simulink model "SVPWM"  (R2026a)
settings: Solver=VariableStepAuto  StopTime=2
undefined symbols (not defined in the file): Down, Up
libraries: eePwmGenerator x3, simulink x3, autolibpmsminterior x2
settings Model: Creator=mushen  LastModifiedBy=mushen

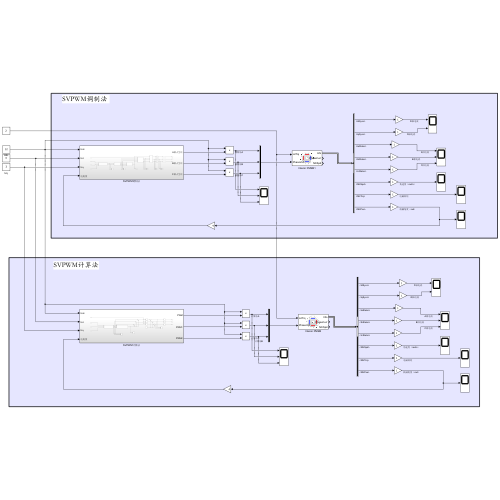
[thumbnail: Simulink's stored preview of the top-level diagram]
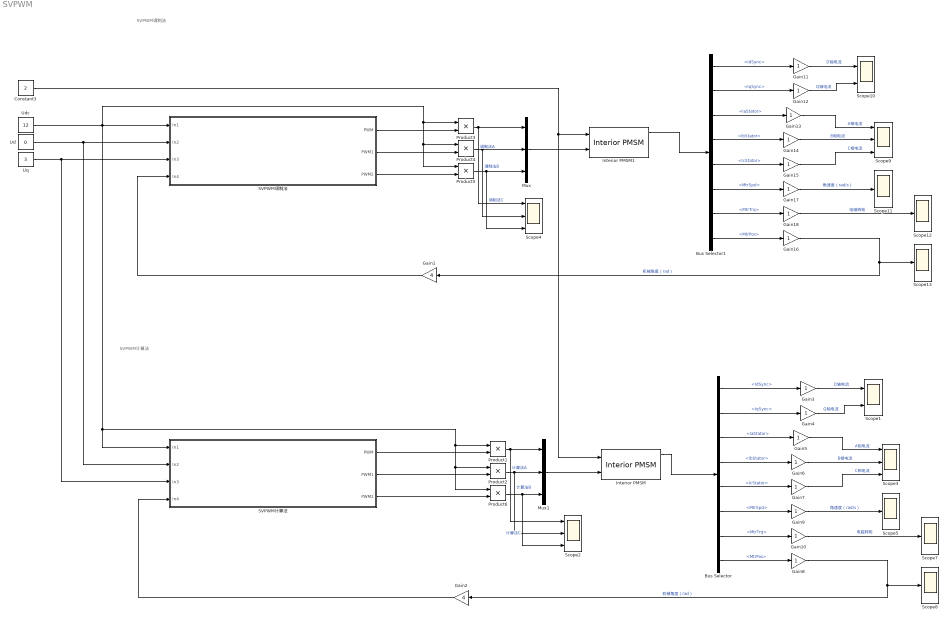
== system SVPWM ==
  note: SVPWM计算法
  note: SVPWM调制法
  Bus Selector : BusSelector  OutputSignals=IdSync,IqSync,IaStator,IbStator,IcStator,MtrSpd,MtrTrq,MtrPos
  Bus Selector1 : BusSelector  OutputSignals=IdSync,IqSync,IaStator,IbStator,IcStator,MtrSpd,MtrTrq,MtrPos
  Constant3 : Constant  Value=2
  Gain1 : Gain  Gain=4
  Gain{3..18} (16 alike) : Gain
  Gain2 : Gain  Gain=4
  Interior PMSM : autolibpmsminterior/Interior PMSM  port_config=Torque  sim_type=Continuous  Ts=0.001  P=4  Rs=0.02  Ldq=[1.7e-3 3.2e-3]  KConstText=Permanent flux linkage constant (lambda_pm):  lambda_pm=0.2205  Ke=159.9771  mechanical=[0.002700,4.924e-4,0]  idq0=[0 0]  theta_init=0  omega_init=0  KConst=0.2205  lambda_pm_calc=0.2205  Kt=0.07  RefBlkName='autolibpmsminterior/Interior PMSM'  aMode=5
      settings: LibrarySourceBlock=mcblib/Electrical Systems/Motors/Interior PMSM
  Interior PMSM1 : autolibpmsminterior/Interior PMSM  port_config=Torque  sim_type=Continuous  Ts=0.001  P=4  Rs=0.02  Ldq=[1.7e-3 3.2e-3]  KConstText=Permanent flux linkage constant (lambda_pm):  lambda_pm=0.2205  Ke=159.9771  mechanical=[0.002700,4.924e-4,0]  idq0=[0 0]  theta_init=0  omega_init=0  KConst=0.2205  lambda_pm_calc=0.2205  Kt=0.07  RefBlkName='autolibpmsminterior/Interior PMSM'  aMode=5
      settings: LibrarySourceBlock=mcblib/Electrical Systems/Motors/Interior PMSM
  Mux : Mux  Inputs=3
  Mux1 : Mux  Inputs=3
  Product{1..6} (6 alike) : Product
  SVPWM计算法 : Subsystem
  SVPWM调制法 : Subsystem
  Scope1 : Scope  NumInputPorts=2
      settings: ActiveDisplayYMinimum=-7.4999999999542695  ActiveDisplayYMaximum=7.49999999991693
  Scope10 : Scope  NumInputPorts=2
      settings: ActiveDisplayYMinimum=-7.4999999999542695  ActiveDisplayYMaximum=7.49999999991693  DataLoggingVariableName=ScopeData15
  Scope{5,7..8,11..13} (6 alike) : Scope
      Scope11 settings: ActiveDisplayYMinimum=-8.3500269440904287  ActiveDisplayYMaximum=20.77178175547505  DataLoggingVariableName=ScopeData16
      Scope12 settings: ActiveDisplayYMinimum=-7.4999999999542695  ActiveDisplayYMaximum=7.49999999991693  DataLoggingVariableName=ScopeData18
      Scope13 settings: ActiveDisplayYMinimum=-7.4999999999542695  ActiveDisplayYMaximum=7.49999999991693  DataLoggingVariableName=ScopeData19
      Scope5 settings: ActiveDisplayYMinimum=-8.3500269440904287  ActiveDisplayYMaximum=20.77178175547505  DataLoggingVariableName=ScopeData10
      Scope7 settings: ActiveDisplayYMinimum=-7.4999999999542695  ActiveDisplayYMaximum=7.49999999991693  DataLoggingVariableName=ScopeData11
      Scope8 settings: ActiveDisplayYMinimum=-7.4999999999542695  ActiveDisplayYMaximum=7.49999999991693  DataLoggingVariableName=ScopeData13
  Scope{2..4,9} (4 alike) : Scope  NumInputPorts=3
      Scope2 settings: ActiveDisplayYMinimum=2.752404735808355  ActiveDisplayYMaximum=9.247595264191645  DataLoggingVariableName=ScopeData8
      Scope3 settings: ActiveDisplayYMinimum=-42.298704643275528  ActiveDisplayYMaximum=42.305828836843332  DataLoggingVariableName=ScopeData9
      Scope4 settings: ActiveDisplayYMinimum=2.752404735808355  ActiveDisplayYMaximum=9.247595264191645  DataLoggingVariableName=ScopeData12
      Scope9 settings: ActiveDisplayYMinimum=-4.8189262546367582  ActiveDisplayYMaximum=4.9055197474515557  DataLoggingVariableName=ScopeData20
  Ud : Constant  Value=0
  Udc : Constant  Value=12
  Uq : Constant  Value=3
  wires:
  SVPWM调制法/1(PWM) -> Product3/2
  Product2/1 -> Scope2/2, Mux1/2  "计算法B"
  Uq/1 -> SVPWM计算法/3(In3), SVPWM调制法/3(In3)
  Udc/1 -> Product2/1, Product6/1, Product1/1, SVPWM计算法/1(In1), Product4/1, Product5/1, Product3/1, SVPWM调制法/1(In1)
  SVPWM计算法/3(PWM2) -> Product6/2
  Product6/1 -> Scope2/3, Mux1/3  "计算法C"
  Product1/1 -> Scope2/1, Mux1/1  "计算法A"
  SVPWM计算法/1(PWM) -> Product1/2
  Gain1/1 -> SVPWM调制法/4(In4)
  Product3/1 -> Scope4/1, Mux/1  "调制法A"
  Ud/1 -> SVPWM计算法/2(In2), SVPWM调制法/2(In2)
  SVPWM调制法/3(PWM2) -> Product5/2
  Gain2/1 -> SVPWM计算法/4(In4)
  SVPWM计算法/2(PWM1) -> Product2/2
  SVPWM调制法/2(PWM1) -> Product4/2
  Product5/1 -> Mux/3, Scope4/3  "调制法C"
  Product4/1 -> Scope4/2, Mux/2  "调制法B"
  Mux1/1 -> Interior PMSM/2
  Mux/1 -> Interior PMSM1/2
  Bus Selector/6 -> Gain9/1  "<MtrSpd>"
  Bus Selector/4 -> Gain6/1  "<IbStator>"
  Bus Selector/5 -> Gain7/1  "<IcStator>"
  Bus Selector/3 -> Gain5/1  "<IaStator>"
  Gain4/1 -> Scope1/2  "Q轴电流"
  Bus Selector/8 -> Gain8/1  "<MtrPos>"
  Bus Selector/1 -> Gain3/1  "<IdSync>"
  Gain3/1 -> Scope1/1  "D轴电流"
  Gain9/1 -> Scope5/1  "角速度（rad/s）"
  Gain6/1 -> Scope3/2  "B相电流"
  Gain7/1 -> Scope3/3  "C相电流"
  Bus Selector/2 -> Gain4/1  "<IqSync>"
  Gain10/1 -> Scope7/1  "电磁转矩"
  Bus Selector/7 -> Gain10/1  "<MtrTrq>"
  Interior PMSM/1 -> Bus Selector/1
  Gain5/1 -> Scope3/1  "A相电流"
  Gain8/1 -> Gain2/1, Scope8/1  "机械角度（rad）"
  Bus Selector1/6 -> Gain17/1  "<MtrSpd>"
  Bus Selector1/4 -> Gain14/1  "<IbStator>"
  Bus Selector1/5 -> Gain15/1  "<IcStator>"
  Bus Selector1/3 -> Gain13/1  "<IaStator>"
  Gain12/1 -> Scope10/2  "Q轴电流"
  Bus Selector1/8 -> Gain16/1  "<MtrPos>"
  Bus Selector1/1 -> Gain11/1  "<IdSync>"
  Gain11/1 -> Scope10/1  "D轴电流"
  Gain17/1 -> Scope11/1  "角速度（rad/s）"
  Gain14/1 -> Scope9/2  "B相电流"
  Gain15/1 -> Scope9/3  "C相电流"
  Bus Selector1/2 -> Gain12/1  "<IqSync>"
  Gain18/1 -> Scope12/1  "电磁转矩"
  Bus Selector1/7 -> Gain18/1  "<MtrTrq>"
  Gain13/1 -> Scope9/1  "A相电流"
  Gain16/1 -> Gain1/1, Scope13/1  "机械角度（rad）"
  Interior PMSM1/1 -> Bus Selector1/1
  Constant3/1 -> Interior PMSM/1, Interior PMSM1/1

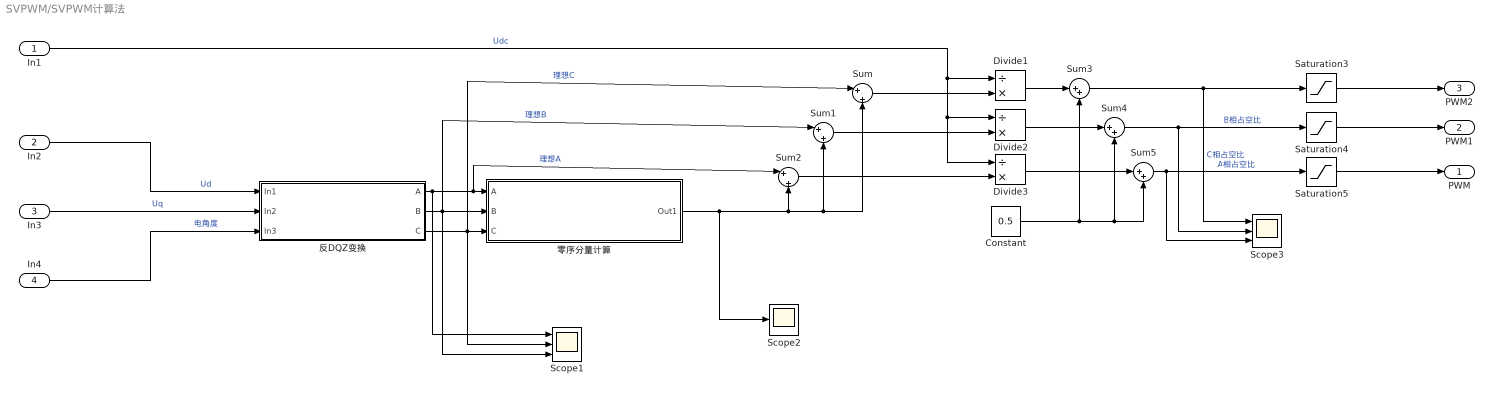
== system SVPWM/SVPWM计算法 ==
  In1 : Inport
  In2 : Inport  Port=2
  In3 : Inport  Port=3
  In4 : Inport  Port=4
  Constant : Constant  Value=0.5
  Divide1 : Product  Inputs=/*
  Divide2 : Product  Inputs=/*
  Divide3 : Product  Inputs=/*
  Saturation3 : Saturate  UpperLimit=1  LowerLimit=0
  Saturation4 : Saturate  UpperLimit=1  LowerLimit=0
  Saturation5 : Saturate  UpperLimit=1  LowerLimit=0
  Scope1 : Scope  NumInputPorts=3
      settings: ActiveDisplayYMinimum=-3.13505  ActiveDisplayYMaximum=3.34432  DataLoggingVariableName=ScopeData2
  Scope2 : Scope
      settings: ActiveDisplayYMinimum=-0.20463  ActiveDisplayYMaximum=-0.00463  DataLoggingVariableName=ScopeData4
  Scope3 : Scope  NumInputPorts=3
      settings: ActiveDisplayYMinimum=0.23003  ActiveDisplayYMaximum=0.76997  DataLoggingVariableName=ScopeData3
  Sum : Sum  Inputs=|+|+
  Sum1 : Sum  Inputs=|+|+
  Sum2 : Sum  Inputs=|+|+
  Sum3 : Sum  Inputs=|++
  Sum4 : Sum  Inputs=|++
  Sum5 : Sum  Inputs=|++
  反DQZ变换 : Subsystem
  零序分量计算 : Subsystem
  PWM : Outport
  PWM1 : Outport  Port=2
  PWM2 : Outport  Port=3
  wires:
  Sum5/1 -> Scope3/3, Saturation5/1  "A相占空比"
  Sum4/1 -> Saturation4/1, Scope3/2  "B相占空比"
  In3/1 -> 反DQZ变换/2(In2)  "Uq"
  In4/1 -> 反DQZ变换/3(In3)  "电角度"
  Sum3/1 -> Scope3/1, Saturation3/1  "C相占空比"
  In2/1 -> 反DQZ变换/1(In1)  "Ud"
  反DQZ变换/1(A) -> Sum2/1, 零序分量计算/1(A), Scope1/1  "理想A"
  反DQZ变换/2(B) -> Sum1/1, Scope1/3, 零序分量计算/2(B)  "理想B"
  反DQZ变换/3(C) -> Sum/1, Scope1/2, 零序分量计算/3(C)  "理想C"
  零序分量计算/1(Out1) -> Sum2/2, Sum/2, Sum1/2, Scope2/1
  Sum2/1 -> Divide3/2
  Sum1/1 -> Divide2/2
  Sum/1 -> Divide1/2
  In1/1 -> Divide3/1, Divide2/1, Divide1/1  "Udc"
  Divide1/1 -> Sum3/1
  Divide3/1 -> Sum5/1
  Divide2/1 -> Sum4/1
  Constant/1 -> Sum3/2, Sum4/2, Sum5/2
  Saturation4/1 -> PWM1/1
  Saturation3/1 -> PWM2/1
  Saturation5/1 -> PWM/1

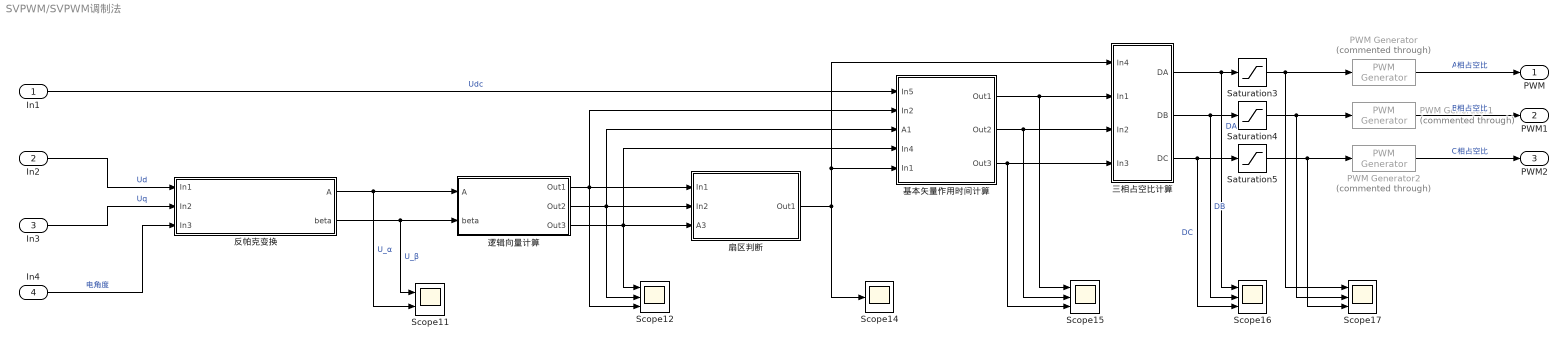
== system SVPWM/SVPWM调制法 ==
  In1 : Inport
  In2 : Inport  Port=2
  In3 : Inport  Port=3
  In4 : Inport  Port=4
  PWM Generator : eePwmGenerator/PWM Generator  Commented=through  CarrCount=Up-Down  Tper=1/16000  Tdelay=0  Ts=5e-6
  PWM Generator1 : eePwmGenerator/PWM Generator  Commented=through  CarrCount=Up-Down  Tper=1/16000  Tdelay=0  Ts=5e-6
  PWM Generator2 : eePwmGenerator/PWM Generator  Commented=through  CarrCount=Up-Down  Tper=1/16000  Tdelay=0  Ts=5e-6
  Saturation3 : Saturate  UpperLimit=1  LowerLimit=0
  Saturation4 : Saturate  UpperLimit=1  LowerLimit=0
  Saturation5 : Saturate  UpperLimit=1  LowerLimit=0
  Scope11 : Scope  NumInputPorts=2
      settings: SampleTime=0.00001  ActiveDisplayYMinimum=-1.82854  ActiveDisplayYMaximum=10.17881
  Scope{12,15..17} (4 alike) : Scope  NumInputPorts=3
      Scope12 settings: ActiveDisplayYMinimum=-6.25  ActiveDisplayYMaximum=6.25  DataLoggingVariableName=ScopeData2
      Scope15 settings: ActiveDisplayYMinimum=-0.09375  ActiveDisplayYMaximum=0.84375  DataLoggingVariableName=ScopeData5
      Scope16 settings: ActiveDisplayYMinimum=0.22937  ActiveDisplayYMaximum=0.77063  DataLoggingVariableName=ScopeData6
      Scope17 settings: ActiveDisplayYMinimum=0.43459  ActiveDisplayYMaximum=1.06282  DataLoggingVariableName=ScopeData7
  Scope14 : Scope
      settings: ActiveDisplayYMinimum=0.375  ActiveDisplayYMaximum=6.625  DataLoggingVariableName=ScopeData4
  三相占空比计算 : Subsystem
  反帕克变换 : Subsystem
  基本矢量作用时间计算 : Subsystem
  扇区判断 : Subsystem
  逻辑向量计算 : Subsystem
  PWM : Outport
  PWM1 : Outport  Port=2
  PWM2 : Outport  Port=3
  wires:
  Saturation4/1 -> PWM Generator1/1, Scope17/2
  逻辑向量计算/2(Out2) -> 基本矢量作用时间计算/3(A1), Scope12/2, 扇区判断/2(In2)
  三相占空比计算/3(DC) -> Scope16/3, Saturation5/1  "DC"
  PWM Generator/1 -> PWM/1  "A相占空比"
  基本矢量作用时间计算/1(Out1) -> 三相占空比计算/2(In1), Scope15/1
  反帕克变换/1(A) -> Scope11/2, 逻辑向量计算/1(A)  "U_α"
  基本矢量作用时间计算/3(Out3) -> 三相占空比计算/4(In3), Scope15/3
  基本矢量作用时间计算/2(Out2) -> 三相占空比计算/3(In2), Scope15/2
  Saturation3/1 -> Scope17/1, PWM Generator/1
  扇区判断/1(Out1) -> Scope14/1, 三相占空比计算/1(In4), 基本矢量作用时间计算/5(In1)
  三相占空比计算/2(DB) -> Scope16/2, Saturation4/1  "DB"
  PWM Generator1/1 -> PWM1/1  "B相占空比"
  反帕克变换/2(beta) -> Scope11/1, 逻辑向量计算/2(beta)  "U_β"
  三相占空比计算/1(DA) -> Scope16/1, Saturation3/1  "DA"
  Saturation5/1 -> PWM Generator2/1, Scope17/3
  逻辑向量计算/1(Out1) -> 扇区判断/1(In1), 基本矢量作用时间计算/2(In2), Scope12/3
  逻辑向量计算/3(Out3) -> 基本矢量作用时间计算/4(In4), Scope12/1, 扇区判断/3(A3)
  In3/1 -> 反帕克变换/2(In2)  "Uq"
  In4/1 -> 反帕克变换/3(In3)  "电角度"
  PWM Generator2/1 -> PWM2/1  "C相占空比"
  In1/1 -> 基本矢量作用时间计算/1(In5)  "Udc"
  In2/1 -> 反帕克变换/1(In1)  "Ud"

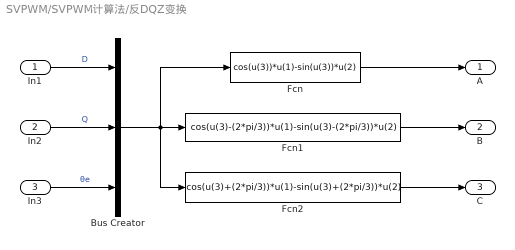
== system SVPWM/SVPWM计算法/反DQZ变换 ==
  In1 : Inport
  In2 : Inport  Port=2
  In3 : Inport  Port=3
  Bus Creator : BusCreator  Inputs=3
  Fcn : Fcn  Expr=cos(u(3))*u(1)-sin(u(3))*u(2)
  Fcn1 : Fcn  Expr=cos(u(3)-(2*pi/3))*u(1)-sin(u(3)-(2*pi/3))*u(2)
  Fcn2 : Fcn  Expr=cos(u(3)+(2*pi/3))*u(1)-sin(u(3)+(2*pi/3))*u(2)
  A : Outport
  B : Outport  Port=2
  C : Outport  Port=3
  wires:
  In3/1 -> Bus Creator/3  "θe"
  In2/1 -> Bus Creator/2  "Q"
  In1/1 -> Bus Creator/1  "D"
  Bus Creator/1 -> Fcn/1, Fcn1/1, Fcn2/1
  Fcn/1 -> A/1
  Fcn1/1 -> B/1
  Fcn2/1 -> C/1

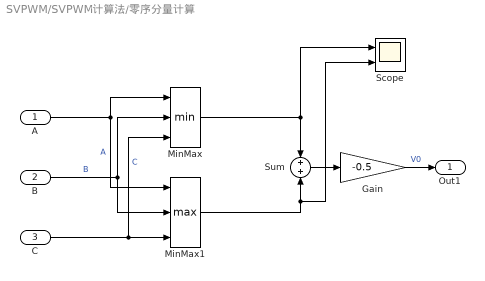
== system SVPWM/SVPWM计算法/零序分量计算 ==
  A : Inport
  B : Inport  Port=2
  C : Inport  Port=3
  Gain : Gain  Gain=-0.5
  MinMax : MinMax  Inputs=3
  MinMax1 : MinMax  Function=max  Inputs=3
  Scope : Scope  NumInputPorts=2
      settings: ActiveDisplayYMinimum=-3.75  ActiveDisplayYMaximum=3.75  DataLoggingVariableName=ScopeData3
  Sum : Sum
  Out1 : Outport
  wires:
  A/1 -> MinMax/1, MinMax1/1  "A"
  B/1 -> MinMax1/2, MinMax/2  "B"
  C/1 -> MinMax/3, MinMax1/3  "C"
  MinMax/1 -> Sum/1, Scope/1
  MinMax1/1 -> Scope/2, Sum/2
  Sum/1 -> Gain/1
  Gain/1 -> Out1/1  "V0"

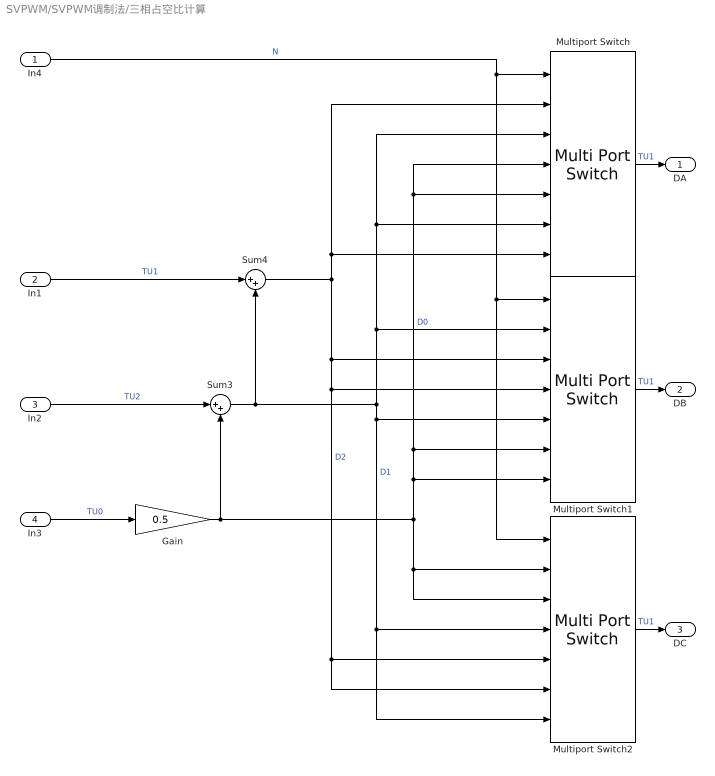
== system SVPWM/SVPWM调制法/三相占空比计算 ==
  In4 : Inport
  In1 : Inport  Port=2
  In2 : Inport  Port=3
  In3 : Inport  Port=4
  Gain : Gain  Gain=0.5
  Multiport Switch : MultiPortSwitch  Inputs=6  SaturateOnIntegerOverflow=off  InputSameDT=off
  Multiport Switch1 : MultiPortSwitch  Inputs=6  SaturateOnIntegerOverflow=off  InputSameDT=off
  Multiport Switch2 : MultiPortSwitch  Inputs=6  SaturateOnIntegerOverflow=off  InputSameDT=off
  Sum3 : Sum  Inputs=|++
  Sum4 : Sum  Inputs=|++
  DA : Outport
  DB : Outport  Port=2
  DC : Outport  Port=3
  wires:
  Multiport Switch/1 -> DA/1  "TU1"
  Multiport Switch1/1 -> DB/1  "TU1"
  Multiport Switch2/1 -> DC/1  "TU1"
  In3/1 -> Gain/1  "TU0"
  In2/1 -> Sum3/1  "TU2"
  Sum3/1 -> Multiport Switch2/7, Multiport Switch2/4, Multiport Switch1/5, Multiport Switch1/2, Multiport Switch/3, Multiport Switch/6, Sum4/2  "D1"
  In1/1 -> Sum4/1  "TU1"
  In4/1 -> Multiport Switch/1, Multiport Switch1/1, Multiport Switch2/1  "N"
  Sum4/1 -> Multiport Switch2/6, Multiport Switch2/5, Multiport Switch1/4, Multiport Switch1/3, Multiport Switch/7, Multiport Switch/2  "D2"
  Gain/1 -> Multiport Switch1/7, Multiport Switch/5, Multiport Switch/4, Multiport Switch1/6, Multiport Switch2/2, Multiport Switch2/3, Sum3/2  "D0"

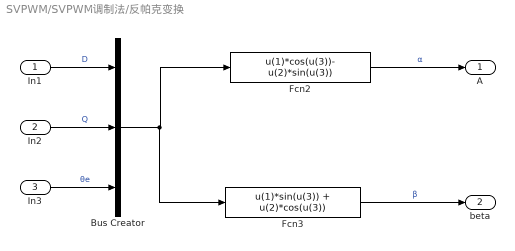
== system SVPWM/SVPWM调制法/反帕克变换 ==
  In1 : Inport
  In2 : Inport  Port=2
  In3 : Inport  Port=3
  Bus Creator : BusCreator  Inputs=3
  Fcn2 : Fcn  Expr=u(1)*cos(u(3))- u(2)*sin(u(3))
  Fcn3 : Fcn  Expr=u(1)*sin(u(3)) + u(2)*cos(u(3))
  A : Outport
  beta : Outport  Port=2
  wires:
  In3/1 -> Bus Creator/3  "θe"
  In2/1 -> Bus Creator/2  "Q"
  In1/1 -> Bus Creator/1  "D"
  Bus Creator/1 -> Fcn2/1, Fcn3/1
  Fcn3/1 -> beta/1  "β"
  Fcn2/1 -> A/1  "α"

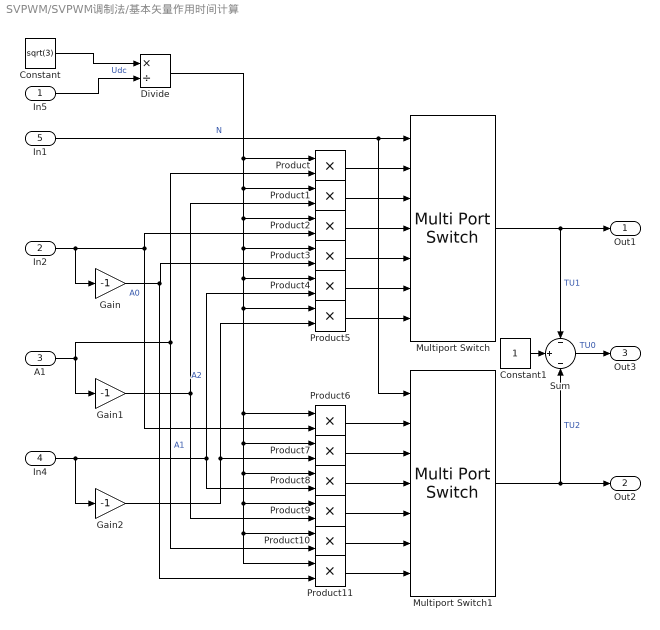
== system SVPWM/SVPWM调制法/基本矢量作用时间计算 ==
  In5 : Inport
  In2 : Inport  Port=2
  A1 : Inport  Port=3
  In4 : Inport  Port=4
  In1 : Inport  Port=5
  Constant : Constant  Value=sqrt(3)
  Constant1 : Constant
  Divide : Product  Inputs=*/
  Gain : Gain  Gain=-1
  Gain1 : Gain  Gain=-1
  Gain2 : Gain  Gain=-1
  Multiport Switch : MultiPortSwitch  Inputs=6  SaturateOnIntegerOverflow=off  InputSameDT=off
  Multiport Switch1 : MultiPortSwitch  Inputs=6  SaturateOnIntegerOverflow=off  InputSameDT=off
  Product{,1..11} (12 alike) : Product
  Sum : Sum  Inputs=-|+|-
  Out1 : Outport
  Out2 : Outport  Port=2
  Out3 : Outport  Port=3
  wires:
  In1/1 -> Multiport Switch1/1, Multiport Switch/1  "N"
  Multiport Switch1/1 -> Sum/3, Out2/1  "TU2"
  Multiport Switch/1 -> Sum/1, Out1/1  "TU1"
  In5/1 -> Divide/2  "Udc"
  Constant/1 -> Divide/1
  Product/1 -> Multiport Switch/2
  Product5/1 -> Multiport Switch/7
  Product4/1 -> Multiport Switch/6
  Product3/1 -> Multiport Switch/5
  Product2/1 -> Multiport Switch/4
  Product1/1 -> Multiport Switch/3
  Divide/1 -> Product/1, Product6/1, Product11/1, Product10/1, Product9/1, Product8/1, Product7/1, Product5/1, Product4/1, Product3/1, Product2/1, Product1/1
  Product6/1 -> Multiport Switch1/2
  Product7/1 -> Multiport Switch1/3
  Product8/1 -> Multiport Switch1/4
  Product9/1 -> Multiport Switch1/5
  Product10/1 -> Multiport Switch1/6
  Product11/1 -> Multiport Switch1/7
  In2/1 -> Gain/1, Product6/2, Product2/2  "A0"
  A1/1 -> Product10/2, Product/2, Gain1/1  "A1"
  In4/1 -> Product4/2, Product8/2, Gain2/1  "A2"
  Gain1/1 -> Product9/2, Product1/2
  Gain/1 -> Product11/2, Product3/2
  Gain2/1 -> Product7/2, Product5/2
  Sum/1 -> Out3/1  "TU0"
  Constant1/1 -> Sum/2

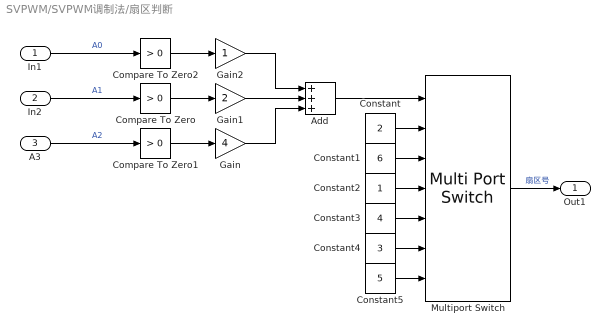
== system SVPWM/SVPWM调制法/扇区判断 ==
  In1 : Inport
  In2 : Inport  Port=2
  A3 : Inport  Port=3
  Add : Sum  Inputs=+++
  Compare To Zero : simulink/Logic and Bit Operations/Compare To Zero  relop=>  OutDataTypeStr=boolean
  Compare To Zero1 : simulink/Logic and Bit Operations/Compare To Zero  relop=>  OutDataTypeStr=boolean
  Compare To Zero2 : simulink/Logic and Bit Operations/Compare To Zero  relop=>  OutDataTypeStr=boolean
  Constant : Constant  Value=2
  Constant1 : Constant  Value=6
  Constant2 : Constant
  Constant3 : Constant  Value=4
  Constant4 : Constant  Value=3
  Constant5 : Constant  Value=5
  Gain : Gain  Gain=4
  Gain1 : Gain  Gain=2
  Gain2 : Gain
  Multiport Switch : MultiPortSwitch  Inputs=6  SaturateOnIntegerOverflow=off  InputSameDT=off
  Out1 : Outport
  wires:
  In1/1 -> Compare To Zero2/1  "A0"
  In2/1 -> Compare To Zero/1  "A1"
  A3/1 -> Compare To Zero1/1  "A2"
  Compare To Zero2/1 -> Gain2/1
  Compare To Zero/1 -> Gain1/1
  Compare To Zero1/1 -> Gain/1
  Gain2/1 -> Add/1
  Gain1/1 -> Add/2
  Gain/1 -> Add/3
  Add/1 -> Multiport Switch/1
  Constant/1 -> Multiport Switch/2
  Constant1/1 -> Multiport Switch/3
  Constant2/1 -> Multiport Switch/4
  Constant3/1 -> Multiport Switch/5
  Constant4/1 -> Multiport Switch/6
  Constant5/1 -> Multiport Switch/7
  Multiport Switch/1 -> Out1/1  "扇区号"

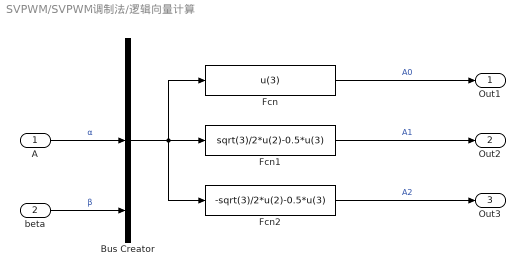
== system SVPWM/SVPWM调制法/逻辑向量计算 ==
  A : Inport
  beta : Inport  Port=2
  Bus Creator : BusCreator  Inputs=3
  Fcn : Fcn  Expr=u(3)
  Fcn1 : Fcn  Expr=sqrt(3)/2*u(2)-0.5*u(3)
  Fcn2 : Fcn  Expr=-sqrt(3)/2*u(2)-0.5*u(3)
  Out1 : Outport
  Out2 : Outport  Port=2
  Out3 : Outport  Port=3
  wires:
  A/1 -> Bus Creator/2  "α"
  beta/1 -> Bus Creator/3  "β"
  ? -> Bus Creator/1  "U_dc"
  Bus Creator/1 -> Fcn2/1, Fcn1/1, Fcn/1
  Fcn/1 -> Out1/1  "A0"
  Fcn1/1 -> Out2/1  "A1"
  Fcn2/1 -> Out3/1  "A2"
